simulink model "TripComputerAlgoLib"  (R2018b)
settings: Solver=VariableStepAuto  StartTime=0.0  StopTime=10.0  RelTol=1e-3
settings Model: Creator=beniamin.costandin  LastModifiedBy=beniamin.costandin

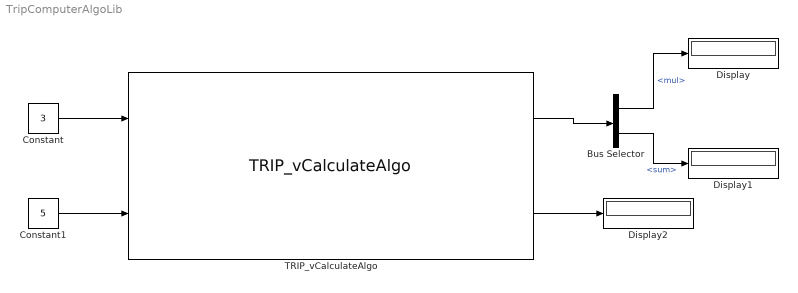
== system TripComputerAlgoLib ==
  Bus Selector : BusSelector  OutputSignals=mul,sum
  Constant : Constant  Value=3  OutDataTypeStr=uint8
  Constant1 : Constant  Value=5  OutDataTypeStr=uint8
  Display : Display
  Display1 : Display
  Display2 : Display
  TRIP_vCalculateAlgo : S-Function  FunctionName=TRIP_vCalculateAlgo  SFunctionDeploymentMode=off  EnableBusSupport=off  mask(Legacy Function){SFunctionSpec=TRIP__tstData y1 = TRIP_vCalculateAlgo(uint8 y2[1], uint8 u1, uint8 u2), ShowSpec=on}
      mask prompts: ShowSpec "Display function specification"
      mask help:
      | This block allows you to call the legacy functions specified by the following Legacy Code Tool definition:
      | def.SFunctionName = 'TRIP_vCalculateAlgo';
      | def.OutputFcnSpec = 'TRIP__tstData y1 = TRIP_vCalculateAlgo(uint8 y2[1], uint8 u1, uint8 u2)';
      | def.HeaderFiles = {'trip.h'};
      | def.SourceFiles = {'trip.c'};
      | def.IncPaths = {'in\inc'};
      mask Help: <p>This block was generated automatically by the Legacy Code Tool. For detailed help on this tool, call<a href="matlab:legacy_code('help')"> legacy_code('help')</a>.</p>
      mask Callback ShowSpec:
      | if strcmp(get_param(gcbh, 'ShowSpec'), 'on')
      |   set_param(gcbh, 'MaskDisplay', sprintf('fprintf(''%s'');', get_param(gcbh, 'SFunctionSpec')));
      | else
      |   set_param(gcbh, 'MaskDisplay', sprintf('fprintf(''%s'');', get_param(gcbh, 'FunctionName')));
      | end
      mask Display: fprintf('TRIP__tstData y1 = TRIP_vCalculateAlgo(uint8 y2[1], uint8 u1, uint8 u2)');
  wires:
  Constant1/1 -> TRIP_vCalculateAlgo/2
  Constant/1 -> TRIP_vCalculateAlgo/1
  TRIP_vCalculateAlgo/1 -> Bus Selector/1
  Bus Selector/1 -> Display/1  "<mul>"
  Bus Selector/2 -> Display1/1  "<sum>"
  TRIP_vCalculateAlgo/2 -> Display2/1
